simulink model "sinus"  (R2022b)
settings: Solver=FixedStepAuto  StartTime=0.0  StopTime=100  FixedStep=0.01  MaxStep=0.01  MinStep=0.01  RelTol=1e-3
settings Model: Creator=wojna  LastModifiedBy=wojna
settings SolverCC: InitialStep=0.01

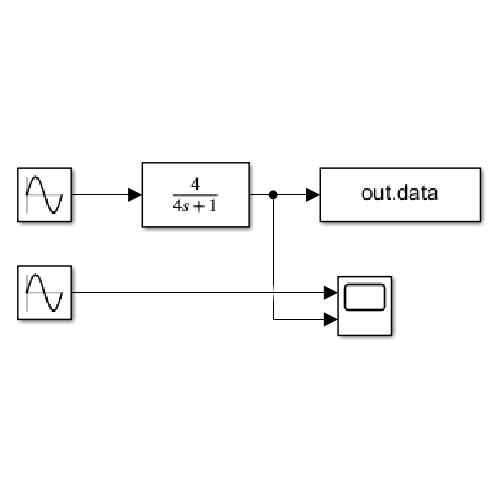
[thumbnail: Simulink's stored preview of the top-level diagram]
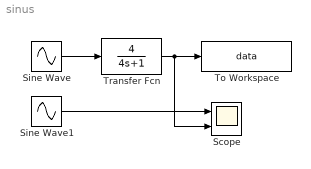
== system sinus ==
  Scope : Scope  NumInputPorts=2
  Sine Wave : Sin  Frequency=0.35  SampleTime=0
  Sine Wave1 : Sin  Frequency=0.35  SampleTime=0
  To Workspace : ToWorkspace  VariableName=data  SaveFormat=Timeseries  SampleTime=-1
  Transfer Fcn : TransferFcn  Numerator=[4]  Denominator=[4 1]
  wires:
  Sine Wave/1 -> Transfer Fcn/1
  Transfer Fcn/1 -> Scope/2, To Workspace/1
  Sine Wave1/1 -> Scope/1
